simulink model "t2_simulink"  (R2018b)
settings: Solver=VariableStepAuto  StartTime=0.0  StopTime=10.0  RelTol=1e-3
libraries: simulink x1
settings Model: Creator=Talha  LastModifiedBy=Talha

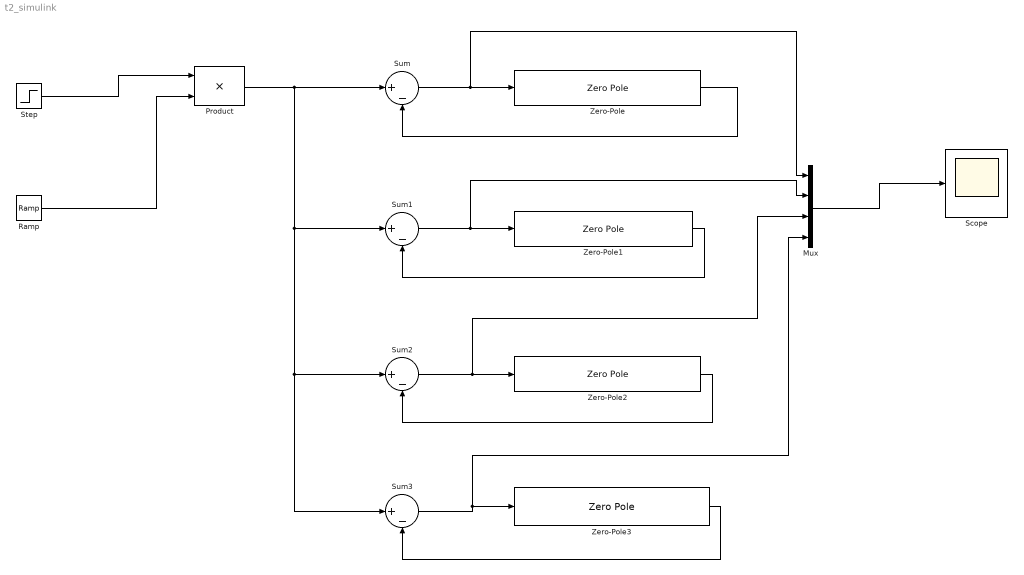
== system t2_simulink ==
  Mux : Mux
  Product : Product
  Ramp : simulink/Sources/Ramp  slope=1  start=0  InitialOutput=0
  Scope : Scope
  Step : Step  After=5  SampleTime=0
  Sum{,1..3} (4 alike) : Sum  Inputs=|+-
  Zero-Pole : ZeroPole  Zeros=[-6]  Poles=[-4 -7 -9 -12]  Gain=[50]
  Zero-Pole1 : ZeroPole  Zeros=[-6]  Poles=[-4 -7 -9 -12]  Gain=[500]
  Zero-Pole2 : ZeroPole  Zeros=[-6]  Poles=[-4 -7 -9 -12]  Gain=[1000]
  Zero-Pole3 : ZeroPole  Zeros=[-6]  Poles=[-4 -7 -9 -12]  Gain=[5000]
  wires:
  Mux/1 -> Scope/1
  Sum3/1 -> Mux/4, Zero-Pole3/1
  Zero-Pole1/1 -> Sum1/2
  Zero-Pole/1 -> Sum/2
  Product/1 -> Sum3/1, Sum2/1, Sum1/1, Sum/1
  Sum1/1 -> Zero-Pole1/1, Mux/2
  Zero-Pole3/1 -> Sum3/2
  Zero-Pole2/1 -> Sum2/2
  Sum/1 -> Zero-Pole/1, Mux/1
  Sum2/1 -> Zero-Pole2/1, Mux/3
  Step/1 -> Product/1
  Ramp/1 -> Product/2
